simulink model "Scatola1"  (R2019a)
settings: Solver=VariableStepAuto  StartTime=0.0  StopTime=10.0  RelTol=1e-3
settings Model: Creator=anton  LastModifiedBy=anton

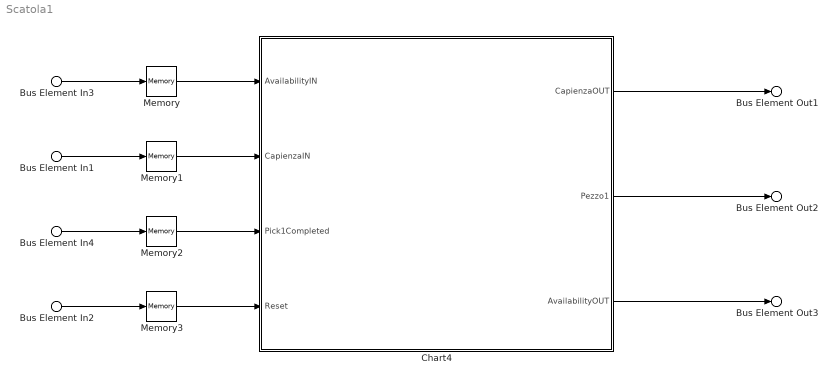
== system Scatola1 ==
  Bus Element In1 : Inport  PortName=CapienzaIN
  Bus Element In2 : Inport  Port=2  PortName=Reset
  Bus Element In3 : Inport  Port=3  PortName=AvailabilityIN
  Bus Element In4 : Inport  Port=4  PortName=Pick1Completed
  Chart4 : Stateflow chart  BlockKeywords=__PRM__SERIALIZED__DATA__:Stateflow Chart,Stateflow Diagram  TreatAsAtomicUnit=on
  Memory{,1..3} (4 alike) : Memory
  Bus Element Out1 : Outport  PortName=Capienza1OUT
  Bus Element Out2 : Outport  Port=2  PortName=AvailabilityOUT
  Bus Element Out3 : Outport  Port=3  PortName=Pezzo1
  wires:
  Chart4/1(CapienzaOUT) -> Bus Element Out1/1
  Chart4/2(Pezzo1) -> Bus Element Out2/1
  Chart4/3(AvailabilityOUT) -> Bus Element Out3/1
  Bus Element In3/1 -> Memory/1
  Memory/1 -> Chart4/1(AvailabilityIN)
  Bus Element In1/1 -> Memory1/1
  Memory1/1 -> Chart4/2(CapienzaIN)
  Bus Element In4/1 -> Memory2/1
  Memory2/1 -> Chart4/3(Pick1Completed)
  Bus Element In2/1 -> Memory3/1
  Memory3/1 -> Chart4/4(Reset)

== stateflow chart Scatola1/Chart4 ==
  state Idle
    CapienzaOUT=2;
    AvailabilityOUT=AvailabilityIN;
    pause(0.1);
  state Capienza2
    CapienzaOUT=2;
    Pezzo1=1;
    AvailabilityOUT=AvailabilityIN;
    pause(0.1);
  state Waiting
  state Capienza1
    CapienzaOUT=1;
    Pezzo1=1;
    AvailabilityOUT=AvailabilityIN;
    pause(0.1);
  state Waiting1
  state Capienza0
    CapienzaOUT=0;
    Pezzo1=0;
    AvailabilityOUT=AvailabilityIN;
    pause(0.1);
  (default) -> Idle
  Capienza0 -> Idle : [CapienzaIN==1]
  Idle -> Capienza2
  Capienza2 -> Waiting : [Pick1Completed==1]
  Waiting -> Capienza1 : [Reset==1]
  Capienza1 -> Waiting1 : [Pick1Completed==1]
  Waiting1 -> Capienza0 : [Reset==1]
  data: AvailabilityIN input; CapienzaOUT output; Pezzo1 output; AvailabilityOUT output; CapienzaIN input; Pick1Completed input; Reset input
